simulink model "nonlinear_vs_linearized"  (Simulink 8.5)
settings: Solver=ode45  StartTime=0.0  StopTime=1000  RelTol=1e-3
values from neighbouring files (symbols this model uses):
  par_p = 1/400    (= 0.0025)    [nonlinear_vs_linearized_main.m]
  parA = 10    [nonlinear_vs_linearized_main.m]
  parC = 1e-03    (= 0.001)    [nonlinear_vs_linearized_main.m]
  parG = 10    [nonlinear_vs_linearized_main.m]
  parHeq = 5    [nonlinear_vs_linearized_main.m]
  parK1 = -4    [nonlinear_vs_linearized_main.m]
  parK2 = 40    [nonlinear_vs_linearized_main.m]
  parMeq = .25    (= 0.25)    [nonlinear_vs_linearized_main.m]
  parPeq = 5    [nonlinear_vs_linearized_main.m]
undefined symbols (not defined in the file or in its folder): delta_d, delta_r
settings Model: Creator=jag  LastModifiedBy=ACSDC  CovModelRefEnable=off
settings DataIOCC: LimitDataPoints=off  SaveFormat=StructureWithTime
settings OptimizationCC: ExpressionDepthLimit=128
settings DebuggingCC: UnderspecifiedInitializationDetection=Simplified  MergeDetectMultiDrivingBlocksExec=error  FcnCallInpInsideContextMsg=EnableAllAsWarning  StateNameClashWarn=none
settings HardwareCC: ProdIntDivRoundTo=Zero  ProdEndianess=LittleEndian  ProdHWDeviceType=Specified

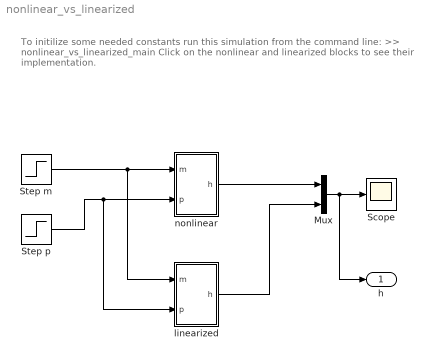
== system nonlinear_vs_linearized ==
  note: To initilize some needed constants run this simulation from the command line:
      | >> nonlinear_vs_linearized_main
      |
      | Click on the nonlinear and linearized blocks to see their implementation.
  Mux : Mux  Inputs=2
  Scope : Scope
      settings: YMin=3.13528  YMax=21.78249
  Step m : Step  Before=parMeq  After=parMeq +delta_d  SampleTime=0
  Step p : Step  Before=parPeq  After=parPeq +delta_r  SampleTime=0
  linearized : Subsystem
  nonlinear : Subsystem
  h : Outport
  wires:
  Step m/1 -> linearized/1(m), nonlinear/1(m)
  Step p/1 -> linearized/2(p), nonlinear/2(p)
  nonlinear/1(h) -> Mux/1
  linearized/1(h) -> Mux/2
  Mux/1 -> h/1, Scope/1

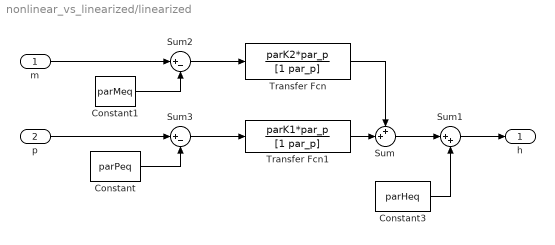
== system nonlinear_vs_linearized/linearized ==
  m : Inport
  p : Inport  Port=2
  Constant : Constant  Value=parPeq
  Constant1 : Constant  Value=parMeq
  Constant3 : Constant  Value=parHeq
  Sum : Sum  Inputs=++|
  Sum1 : Sum  Inputs=|++
  Sum2 : Sum  Inputs=|+-
  Sum3 : Sum  Inputs=|+-
  Transfer Fcn : TransferFcn  Numerator=parK2*par_p  Denominator=[1 par_p]
  Transfer Fcn1 : TransferFcn  Numerator=parK1*par_p  Denominator=[1 par_p]
  h : Outport
  wires:
  Sum1/1 -> h/1
  Constant1/1 -> Sum2/2
  Sum/1 -> Sum1/1
  Sum2/1 -> Transfer Fcn/1
  Constant/1 -> Sum3/2
  Sum3/1 -> Transfer Fcn1/1
  Transfer Fcn/1 -> Sum/1
  p/1 -> Sum3/1
  m/1 -> Sum2/1
  Constant3/1 -> Sum1/2
  Transfer Fcn1/1 -> Sum/2

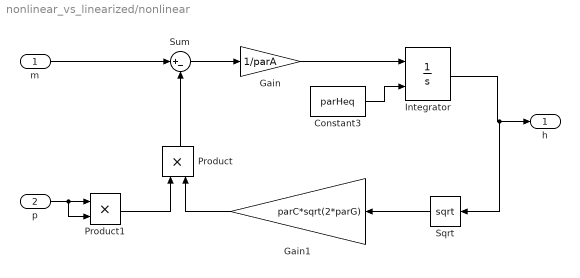
== system nonlinear_vs_linearized/nonlinear ==
  m : Inport
  p : Inport  Port=2
  Constant3 : Constant  Value=parHeq
  Gain : Gain  Gain=1/parA
  Gain1 : Gain  Gain=parC*sqrt(2*parG)
  Integrator : Integrator  InitialConditionSource=external
  Product : Product
  Product1 : Product
  Sqrt : Sqrt  SaturateOnIntegerOverflow=on
  Sum : Sum  Inputs=|+-
  h : Outport
  wires:
  Gain/1 -> Integrator/1
  m/1 -> Sum/1
  Product/1 -> Sum/2
  Sum/1 -> Gain/1
  Gain1/1 -> Product/2
  Sqrt/1 -> Gain1/1
  Integrator/1 -> Sqrt/1, h/1
  Product1/1 -> Product/1
  p/1 -> Product1/2, Product1/1
  Constant3/1 -> Integrator/2
